simulink subsystem "tehrani_alv_mass_balance_co2_integ"  (R2019b)
settings: Solver=VariableStepAuto  StartTime=0.0  StopTime=10.0  RelTol=1e-3
undefined symbols (not defined in the file): __PRM__SERIALIZED__DATA__, SubsystemReferenceBlock
settings Model: Creator=RH  LastModifiedBy=RH

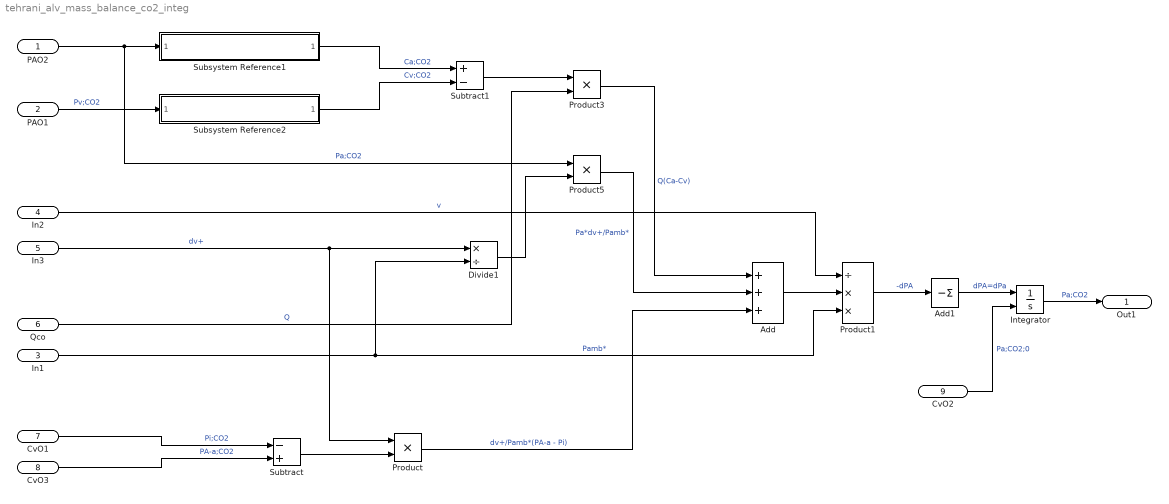
== system tehrani_alv_mass_balance_co2_integ ==
  PAO2 : Inport
  PAO1 : Inport  Port=2
  In1 : Inport  Port=3
  In2 : Inport  Port=4
  In3 : Inport  Port=5
  Qco : Inport  Port=6
  CvO1 : Inport  Port=7
  CvO3 : Inport  Port=8
  CvO2 : Inport  Port=9
  Add : Sum  Inputs=+++
  Add1 : Sum  Inputs=-
  Divide1 : Product  Inputs=*/
  Integrator : Integrator  InitialConditionSource=external
  Product : Product
  Product1 : Product  Inputs=/**
  Product3 : Product
  Product5 : Product
  Subsystem Reference1 : Subsystem  BlockKeywords=__PRM__SERIALIZED__DATA__:SubsystemReferenceBlock  ReferencedSubsystem=CO2_dissociation
  Subsystem Reference2 : Subsystem  BlockKeywords=__PRM__SERIALIZED__DATA__:SubsystemReferenceBlock  ReferencedSubsystem=CO2_dissociation
  Subtract : Sum  Inputs=-+
  Subtract1 : Sum  Inputs=+-
  Out1 : Outport
  wires:
  Product1/1 -> Add1/1  "-dPA"
  In2/1 -> Product1/1  "v"
  Subtract1/1 -> Product3/1
  Subtract/1 -> Product/2
  Divide1/1 -> Product5/2
  Product5/1 -> Add/2  "Pa*dv+/Pamb*"
  Product/1 -> Add/3  "dv+/Pamb*(PA-a - Pi)"
  Add/1 -> Product1/2
  Subsystem Reference2/1 -> Subtract1/2  "Cv;CO2"
  In3/1 -> Divide1/1, Product/1  "dv+"
  Subsystem Reference1/1 -> Subtract1/1  "Ca;CO2"
  In1/1 -> Product1/3, Divide1/2  "Pamb*"
  Qco/1 -> Product3/2  "Q"
  Integrator/1 -> Out1/1  "Pa;CO2"
  Product3/1 -> Add/1  "Q(Ca-Cv)"
  PAO2/1 -> Subsystem Reference1/1, Product5/1  "Pa;CO2"
  CvO1/1 -> Subtract/1  "Pi;CO2"
  CvO3/1 -> Subtract/2  "PA-a;CO2"
  Add1/1 -> Integrator/1  "dPA=dPa"
  PAO1/1 -> Subsystem Reference2/1  "Pv;CO2"
  CvO2/1 -> Integrator/2  "Pa;CO2;0"
